simulink model "ADP_based_triangle_formation_control"  (R2024a)
settings: Solver=VariableStepAuto  StartTime=0.0  StopTime=10  RelTol=1e-3
(part 2 of 2)

== matlab function ADP_based_triangle_formation_control/WMR 1/ADP weight update ==
  data: ep1 input; ep2 input; ep_dot1 input; ep_dot2 input; u_new input; E1 input; E2 input; E3 input; E4 input; W input; d input; alpha input; W_dot output
function W_dot = control(ep1,ep2,ep_dot1,ep_dot2,u_new,E1,E2,E3,E4,W,d,alpha)

lambda = 2;

g_u = [0 0;
       0 0;
       1 0;
       0 1];    % 4x2
g_d = [0 0;
       0 0;
       1 0;
       0 1];    % 4x2

% x1 = ep;
% x2 = ep_dot+lambda*ep;
x11 = ep1;
x12 = ep2;
x21 = ep_dot1+lambda*ep1;
x22 = ep_dot2+lambda*ep2;

% % vec = [x1^2; x1*x2; x2^2];
% % grad_vec = [2*x1 0;      % 3x2
% %             x2 x1;
% %             0 2*x2];
grad_vec = [2*x11 0 0 0;
            0 2*x12 0 0;
            x21 0 x11 0;
            0 x22 0 x12;
            0 0 2*x21 0;
            0 0 0 2*x22];   % 6x4
% 
% x = [x1;x2];   % 4x1
x = [x11;x12;x21;x22];

f = [x21-lambda*x11;
     x22-lambda*x12;
     E1*x21+E3*x22-(E1*lambda*x11+E3*lambda*x12);
     E2*x21+E4*x22-(E2*lambda*x11+E4*lambda*x12)]; 

sig = grad_vec*(f + g_u*u_new + g_d*d);   % 6x1

% Update weights
% alpha1 = 2;
alpha2 = 0.8;
Q = eye(4);
R = eye(2);

% W_dot = (-alpha1*sig*(sig'*W + x'*Q*x + u_new'*R*u_new))/((sig'*sig+1)^2) + (1/2)*alpha2*grad_vec*g_u/R *g_u'*x;

W_dot = -alpha*sig*(sig'*W + x'*Q*x + u_new'*R*u_new) + (1/2)*alpha2*grad_vec*g_u/R *g_u'*x;

end

== matlab function ADP_based_triangle_formation_control/WMR 1/Actual WMR dynamic model ==
  data: wr input; wl input; gamma_r_dd input; gamma_l_dd input; wr_dot output; eta_dot input; eta_dd input; tau input; w input; wl_dot output; dv output; to_right input; to_left input
function [wr_dot,wl_dot,dv]  = Dynamic(wr, wl, gamma_r_dd, gamma_l_dd, eta_dot, eta_dd, tau, w, to_right,to_left)
%% Parameters
mG = 10; %kg
mW = 2; %kg
I_G = 4; %kgm^2
I_W = 0.1; %kgm^2
I_D = 0.05; %kgm^2
a = 0.2; %m
L = 0.6; %m (L=2b)
r = 0.15; %m

m11 = mG*(r^2/4 + a^2*r^2/(L^2)) + r^2*(I_G+2*I_D)/(L^2) + 2*mW*r^2 + I_W;
m12 = mG*(r^2/4 - a^2*r^2/(L^2)) - r^2*(I_G+2*I_D)/(L^2);
m21 = m12;
m22 = m11;
M = [m11 m12;
     m21 m22];
B = mG*a*r^2/L*w*[0 1;-1 0];
Q1 = mG*r*(1+4*a^2/L^2)/4 + r*(I_G+2*I_D)/(2*L);
Q2 = mG*r*(1-4*a^2/L^2)/4 - r*(I_G+2*I_D)/(2*L);
Q = [Q1 Q2;
     Q2 Q1];
C = mG*(r/2)*w*[1;1];
G = mG*(a*r/L)*[1;-1];

gamma_dd = [gamma_r_dd; gamma_l_dd];

%% Dynamics of WMR
V = [wr;wl];
to = [to_right;to_left];
V_dot = (-M\B)*V + M\to - M\(Q*gamma_dd + C*eta_dot + G*eta_dd + tau);

wr_dot = V_dot(1);
wl_dot = V_dot(2);

dv = - M\(Q*gamma_dd + C*eta_dot + G*eta_dd + tau);

end

== matlab function ADP_based_triangle_formation_control/WMR 1/Actual WMR kinematic model  ==
  data: v input; x_dot output; w input; theta input; y_dot output; theta_dot output; S_ output; eta_dot input; dp_ output; gamma_r_dot input; gamma_l_dot input
function [x_dot, y_dot, theta_dot, S_, dp_] = Kinematic (v,w,theta,eta_dot,gamma_r_dot,gamma_l_dot)

L = 0.6; % L =2b
r = 0.15; %m
a = 0.2; %m
% V: Robot velocity matrix
V = [v;w];

S = [cos(theta) -a*sin(theta);
     sin(theta) a*cos(theta);
      0 1];
dp = [-eta_dot*sin(theta);
       eta_dot*cos(theta);
       0];

% V = [wr;wl]
% S = [(r*cos(theta)/2)-(d*r*sin(theta)/L) (r*cos(theta)/2)+(d*r*sin(theta)/L);...
%      (r*sin(theta)/2)+(d*r*cos(theta)/L) (r*sin(theta)/2)-(d*r*cos(theta)/L);...
%       r/L -r/L];
% 
% dp = [(cos(theta)*(gamma_r_dot+gamma_l_dot)/2)-(d*sin(theta)*(gamma_r_dot-gamma_l_dot)/L)-eta_dot*sin(theta);
%       (sin(theta)*(gamma_r_dot+gamma_l_dot)/2)+(d*cos(theta)*(gamma_r_dot-gamma_l_dot)/L)+eta_dot*cos(theta);
%        (gamma_r_dot-gamma_l_dot)/L];

S_ = [(r*cos(theta)/2)-(a*r*sin(theta)/L) (r*cos(theta)/2)+(a*r*sin(theta)/L);
     (r*sin(theta)/2)+(a*r*cos(theta)/L) (r*sin(theta)/2)-(a*r*cos(theta)/L)];

dp_ = [(cos(theta)*(gamma_r_dot+gamma_l_dot)/2)-(a*sin(theta)*(gamma_r_dot-gamma_l_dot)/L)-eta_dot*sin(theta);
      (sin(theta)*(gamma_r_dot+gamma_l_dot)/2)+(a*cos(theta)*(gamma_r_dot-gamma_l_dot)/L)+eta_dot*cos(theta)];

% Output matrix
p_dot = S*V + dp;

% Output value 
x_dot = p_dot(1);
y_dot = p_dot(2);
theta_dot = p_dot(3);

end

== matlab function ADP_based_triangle_formation_control/WMR 1/Control torque ==
  data: u_new input; u input; to_r output; to_l output; S input
function [to_r,to_l] = fcn(u_new, u,S)
mG = 10; %kg
mW = 2; %kg
I_G = 4; %kgm^2
I_W = 0.1; %kgm^2
I_D = 0.05; %kgm^2
a = 0.2; %m
L = 0.6; %m
r = 0.15; %m

m11 = mG*(r^2/4 + a^2*r^2/(L^2)) + r^2*(I_G+2*I_D)/(L^2) + 2*mW*r^2 + I_W;
m12 = mG*(r^2/4 - a^2*r^2/(L^2)) - r^2*(I_G+2*I_D)/(L^2);
m21 = m12;
m22 = m11;
M = [m11 m12;
     m21 m22];

%% S*inv(M)*to-u = u_new
to = (M/S)*(u_new+u);   % to = M*inv(S)*(u_new+u)
to_r = to(1);
to_l = to(2);

end

== matlab function ADP_based_triangle_formation_control/WMR 1/Critic NN ==
  data: eps input; u_new input; E1 input; E2 input; E3 input; E4 input; ep1 input; sig output; ep2 input; ep_dot1 input; ep_dot2 input
function sig  = fcn(eps,u_new,E1,E2,E3,E4,ep1,ep2,ep_dot1,ep_dot2)
lambda = 2;
g_u = [0 0;
       0 0;
       1 0;
       0 1];    % 4x2
g_d = [0 0;
       0 0;
       1 0;
       0 1];    % 4x2

% x1 = ep;
% x2 = ep_dot+lambda*ep;
x11 = ep1;
x12 = ep2;
x21 = ep_dot1+lambda*ep1;
x22 = ep_dot2+lambda*ep2;

% % vec = [x1^2; x1*x2; x2^2];
% % grad_vec = [2*x1 0;      % 3x2
% %             x2 x1;
% %             0 2*x2];
grad_vec = [2*x11 0 0 0;
            0 2*x12 0 0;
            x21 0 x11 0;
            0 x22 0 x12;
            0 0 2*x21 0;
            0 0 0 2*x22];   % 6x4

% f = [x2-lambda*x1; E*x2-E*lambda*x1];   % 4x1
f = [x21-lambda*x11;
     x22-lambda*x12;
     E1*x21+E3*x22-(E1*lambda*x11+E3*lambda*x12);
     E2*x21+E4*x22-(E2*lambda*x11+E4*lambda*x12)]; 
% 
sig = grad_vec*(f + g_u*u_new + g_d*eps);   % 6x1
end

== matlab function ADP_based_triangle_formation_control/WMR 1/Disturbance compensation ==
  data: ep1 input; ep2 input; ep_dot1 input; ep_dot2 input; z input; u_d output; d_observe output
function [u_d, d_observe] = fcn(ep1,ep2,ep_dot1,ep_dot2,z)

lambda = 2;

x11 = ep1;
x12 = ep2;
x21 = ep_dot1+lambda*ep1;
x22 = ep_dot2+lambda*ep2;

% Disturbance observer
x = [x11;x12;x21;x22];
Lf = 30;
eps_ = z + Lf*x;

u_d = -eps_(3:4);

d_observe = eps_(3:4); % for plotting
end

== matlab function ADP_based_triangle_formation_control/WMR 1/Parameters ==
  data: M output; w input; B output; wr input; wl input; v1 input; v2 input; S input; S_dot input; dp input; dp_dot input; dv input; eps1 output; eps2 output
function [M,B,eps1,eps2] = fcn(w,wr,wl,v1,v2,S,S_dot,dp,dp_dot,dv)

mG = 10; %kg
mW = 2; %kg
I_G = 4; %kgm^2
I_W = 0.1; %kgm^2
I_D = 0.05; %kgm^2
a = 0.2; %m
L = 0.6; %m (L=2b)
r = 0.15; %m

m11 = mG*(r^2/4 + a^2*r^2/(L^2)) + r^2*(I_G+2*I_D)/(L^2) + 2*mW*r^2 + I_W;
m12 = mG*(r^2/4 - a^2*r^2/(L^2)) - r^2*(I_G+2*I_D)/(L^2);
m21 = m12;
m22 = m11;
M = [m11 m12;
     m21 m22];
B = mG*a*r^2/L*w*[0 1;-1 0];

V_actual = [wr;wl];
V = [v1;v2];
lambda = 2;

eps1 = dp-V;
eps2 = S*dv + S_dot*V_actual + dp_dot + lambda*S*V_actual + lambda*eps1;
% d = eps2 - E*eps1;    % 2x1

end

== matlab function ADP_based_triangle_formation_control/WMR 1/desired double-integrator WMR model ==
  data: wr input; p_dot1 output; wl input; p_dot2 output; wr_dot output; wl_dot output; u1 input; u2 input
function [p_dot1,p_dot2,wr_dot,wl_dot]  = fcn(wr,wl,u1,u2)
p_dot1 = wr;
p_dot2 = wl;
wr_dot = u1;
wl_dot = u2;

end

== matlab function ADP_based_triangle_formation_control/WMR 1/disturbance observer ==
  data: z input; E1 input; E2 input; E3 input; E4 input; ep1 input; ep2 input; ep_dot1 input; ep_dot2 input; u_new input; z_dot output
function z_dot = fcn(z,E1,E2,E3,E4,ep1,ep2,ep_dot1,ep_dot2,u_new)

lambda = 2;

x11 = ep1;
x12 = ep2;
x21 = ep_dot1+lambda*ep1;
x22 = ep_dot2+lambda*ep2;


% x = [x1;x2];   % 4x1
x = [x11;x12;x21;x22];
% f = [x2-lambda*x1; E*x2-E*lambda*x1];   % 4x1
f = [x21-lambda*x11;
     x22-lambda*x12;
     E1*x21+E3*x22-(E1*lambda*x11+E3*lambda*x12);
     E2*x21+E4*x22-(E2*lambda*x11+E4*lambda*x12)]; 
g_u = [0 0;
       0 0;
       1 0;
       0 1];    % 4x2
g_d = [0;
       0;
       1;
       1];    % 4x1

% Disturbance observer
Lf = 30;   
z_dot = -Lf*(g_d.*(z+Lf*x) + f + g_u*u_new); 

end

== matlab function ADP_based_triangle_formation_control/WMR 1/forward and angular velocity  ==
  data: wr input; v output; wl input; w output; gamma_r_dot input; gamma_l_dot input
function [v,w] = fcn(wr,wl, gamma_r_dot, gamma_l_dot)
L = 0.6; %m (L=2b)
r = 0.15; %m
v = r*(wr+wl)/2 + (gamma_r_dot+gamma_l_dot)/2;
w = r*(wr-wl)/L + (gamma_r_dot-gamma_l_dot)/L;

end

== matlab function ADP_based_triangle_formation_control/WMR 1/p_actual - p ==
  data: x input; ep output; y input; p1 input; p2 input
function ep = error(x,y,p1,p2)
ep1 = x-p1;
ep2 = y-p2;
ep = [ep1;ep2];
end

== matlab function ADP_based_triangle_formation_control/multi-agent tracking control signal ==
  data: uxi output; xi input; yi input; xRef input; yRef input; vx input; vy input; uyi output; ucx input; ucy input
function [uxi,uyi]  = consensus_algo(xi,yi, xRef,yRef, vx,vy, ucx, ucy)
A = [0 0 1;
     1 0 0;
     0 1 0];
D = diag([1, 1, 1]);

alpha1 = 600;
alpha2 = 600;
alpha3 = 600;

Q = diag([alpha1, alpha2, alpha3]);
L = D - A;
% L = [2    -1    -1     0
%     -1     2     0    -1
%      0    -1     1     0
%     -1     0    -1     2]

k1 = 10;
k2 = 120;

% uxi = - k1*(L+Q)*(xi-xRef) - k2*vx;
% uyi = - k1*(L+Q)*(yi-yRef) - k2*vy;

% k = 600;
% uxi = -(k*eye(4)+L)*(xi-xRef) + (-k2*eye(4))*vx;
% uyi = -(k*eye(4)+L)*(yi-yRef) + (-k2*eye(4))*vy;

uxi = -(L+Q)*(xi-xRef) -k2*(vx-ucx);
uyi = -(L+Q)*(yi-yRef) -k2*(vy-ucy);

end

== matlab function ADP_based_triangle_formation_control/desired deviation of robot i w.r.t ref virtual frame ==
  data: xFRef output; yFRef output
function [xFRef, yFRef] = fcn ()
% Triangle formation

l = 0.6;
j = [1;2;3];
% phiRef = pi*[1;1;1;1] - pi/4 * j;
phiRef = 2*pi/3 * (j-1);
xFRef = l*cos(phiRef); 
yFRef = l*sin(phiRef);
          
end

== matlab function ADP_based_triangle_formation_control/reference states (virtual leader)/MATLAB Function ==
  data: x_ref output; y_ref output; theta_ref output; t input
function [x_ref,y_ref,theta_ref] = reference(t)


% Circle trajectory
w = pi/6;
x_ref = 3*sin(w*t);
y_ref = 3*cos(w*t);
dxRef = 3*w*cos(w*t);
dyRef =  -3*w*sin(w*t);
theta_ref =  atan2(dyRef, dxRef);

% Line trajectory
% x_ref = 3+0.75*t;
% y_ref = -2+0.5*t;
% theta_ref = pi;
% dxRef = 0.75;
% dyRef =  0.5;
% theta_ref =  atan2(dyRef, dxRef);

% w = 2*pi/30;
% x_ref = 1.1 + 0.7*sin(w*t);
% y_ref = 0.9 + 0.7*sin(2*w*t);
% dxRef = 0.7*w*cos(w*t);
% dyRef = 1.4*w*cos(2*w*t);
% ddxRef = -0.7*w^2*sin(w*t);
% ddyRef = -2.8*w^2*sin(2*w*t);
% 
% theta_ref =  atan2(dyRef, dxRef);
% 
% v_ref = sqrt(dxRef^2+dyRef^2);
% w_ref = (dxRef*ddyRef-dyRef*ddxRef)/(dxRef^2+dyRef^2);


end

== matlab function ADP_based_triangle_formation_control/robot desired position ==
  data: xRef output; yRef output; xc input; yc input; thetac input; xFRef input; yFRef input
function [xRef, yRef] = fcn (xc, yc, thetac, xFRef, yFRef)
      
xRef = xc + cos(thetac)*xFRef - sin(thetac)*yFRef;
yRef = yc + sin(thetac)*xFRef + cos(thetac)*yFRef;

% xRef = xc + xFRef;
% yRef = yc + yFRef;
end

== matlab function ADP_based_triangle_formation_control/WMR 3/ADP weight update ==
  data: ep1 input; ep2 input; ep_dot1 input; ep_dot2 input; u_new input; E1 input; E2 input; E3 input; E4 input; W input; d input; alpha input; W_dot output
function W_dot = control(ep1,ep2,ep_dot1,ep_dot2,u_new,E1,E2,E3,E4,W,d,alpha)

lambda = 2;

g_u = [0 0;
       0 0;
       1 0;
       0 1];    % 4x2
g_d = [0 0;
       0 0;
       1 0;
       0 1];    % 4x2

% x1 = ep;
% x2 = ep_dot+lambda*ep;
x11 = ep1;
x12 = ep2;
x21 = ep_dot1+lambda*ep1;
x22 = ep_dot2+lambda*ep2;

% % vec = [x1^2; x1*x2; x2^2];
% % grad_vec = [2*x1 0;      % 3x2
% %             x2 x1;
% %             0 2*x2];
grad_vec = [2*x11 0 0 0;
            0 2*x12 0 0;
            x21 0 x11 0;
            0 x22 0 x12;
            0 0 2*x21 0;
            0 0 0 2*x22];   % 6x4
% 
% x = [x1;x2];   % 4x1
x = [x11;x12;x21;x22];

f = [x21-lambda*x11;
     x22-lambda*x12;
     E1*x21+E3*x22-(E1*lambda*x11+E3*lambda*x12);
     E2*x21+E4*x22-(E2*lambda*x11+E4*lambda*x12)]; 

sig = grad_vec*(f + g_u*u_new + g_d*d);   % 6x1

% Update weights
% alpha1 = 2;
alpha2 = 0.8;
Q = eye(4);
R = eye(2);

% W_dot = (-alpha1*sig*(sig'*W + x'*Q*x + u_new'*R*u_new))/((sig'*sig+1)^2) + (1/2)*alpha2*grad_vec*g_u/R *g_u'*x;

W_dot = -alpha*sig*(sig'*W + x'*Q*x + u_new'*R*u_new) + (1/2)*alpha2*grad_vec*g_u/R *g_u'*x;

end

== matlab function ADP_based_triangle_formation_control/WMR 3/Actual WMR dynamic model ==
  data: wr input; wl input; gamma_r_dd input; gamma_l_dd input; wr_dot output; eta_dot input; eta_dd input; tau input; w input; wl_dot output; dv output; to_right input; to_left input
function [wr_dot,wl_dot,dv]  = Dynamic(wr, wl, gamma_r_dd, gamma_l_dd, eta_dot, eta_dd, tau, w, to_right,to_left)
%% Parameters
mG = 10; %kg
mW = 2; %kg
I_G = 4; %kgm^2
I_W = 0.1; %kgm^2
I_D = 0.05; %kgm^2
a = 0.2; %m
L = 0.6; %m (L=2b)
r = 0.15; %m

m11 = mG*(r^2/4 + a^2*r^2/(L^2)) + r^2*(I_G+2*I_D)/(L^2) + 2*mW*r^2 + I_W;
m12 = mG*(r^2/4 - a^2*r^2/(L^2)) - r^2*(I_G+2*I_D)/(L^2);
m21 = m12;
m22 = m11;
M = [m11 m12;
     m21 m22];
B = mG*a*r^2/L*w*[0 1;-1 0];
Q1 = mG*r*(1+4*a^2/L^2)/4 + r*(I_G+2*I_D)/(2*L);
Q2 = mG*r*(1-4*a^2/L^2)/4 - r*(I_G+2*I_D)/(2*L);
Q = [Q1 Q2;
     Q2 Q1];
C = mG*(r/2)*w*[1;1];
G = mG*(a*r/L)*[1;-1];

gamma_dd = [gamma_r_dd; gamma_l_dd];

%% Dynamics of WMR
V = [wr;wl];
to = [to_right;to_left];
V_dot = (-M\B)*V + M\to - M\(Q*gamma_dd + C*eta_dot + G*eta_dd + tau);

wr_dot = V_dot(1);
wl_dot = V_dot(2);

dv = - M\(Q*gamma_dd + C*eta_dot + G*eta_dd + tau);

end
